simulink model "Lab6_StateFB"  (R2016a)
settings: Solver=VariableStepAuto  StartTime=0.0  StopTime=10.0  RelTol=1e-3
settings Model: Creator=jordan  LastModifiedBy=jordan

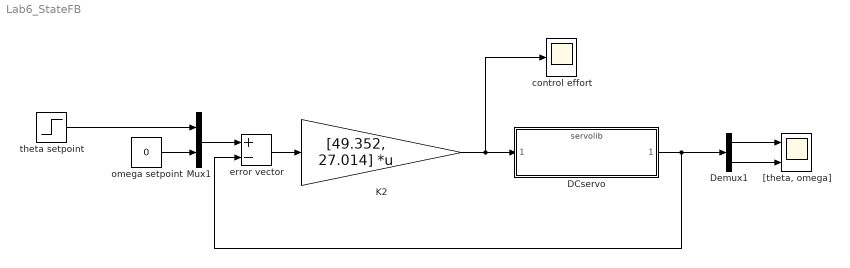
== system Lab6_StateFB ==
  DCservo : ModelReference  ModelNameDialog=servolib.slx  SimulationMode=Normal  ModelReferenceVersion=1.18
  Demux1 : Demux  Outputs=2
  K2 : Gain  Gain=[49.352, 27.014]  Multiplication=Matrix(K*u)
  Mux1 : Mux  Inputs=2
  "[theta, omega]" : Scope  NumInputPorts=2
  control effort : Scope
  error vector : Sum  Inputs=+-
  omega setpoint : Constant  Value=0
  theta setpoint : Step  SampleTime=0
  wires:
  K2/1 -> control effort/1, DCservo/1
  Demux1/1 -> "[theta, omega]"/1
  Demux1/2 -> "[theta, omega]"/2
  omega setpoint/1 -> Mux1/2
  Mux1/1 -> error vector/1
  error vector/1 -> K2/1
  theta setpoint/1 -> Mux1/1
  DCservo/1 -> Demux1/1, error vector/2
